simulink model "Capteur"  (R2019b)
settings: Solver=FixedStepAuto  StartTime=0.0  StopTime=1  FixedStep=0.0001  RelTol=1e-3
settings Model: Creator=Dell XPS  LastModifiedBy=jeanz
settings SolverCC: InitialStep=0.0001

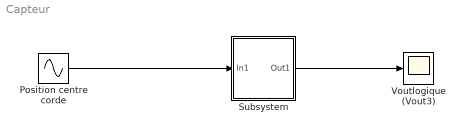
== system Capteur ==
  Position centre corde : Sin  Amplitude=0.1  Bias=2.415  Frequency=1256  SampleTime=0
  Subsystem : Subsystem
  Voutlogique (Vout3) : Scope
  wires:
  Position centre corde/1 -> Subsystem/1(In1)
  Subsystem/1(Out1) -> Voutlogique (Vout3)/1

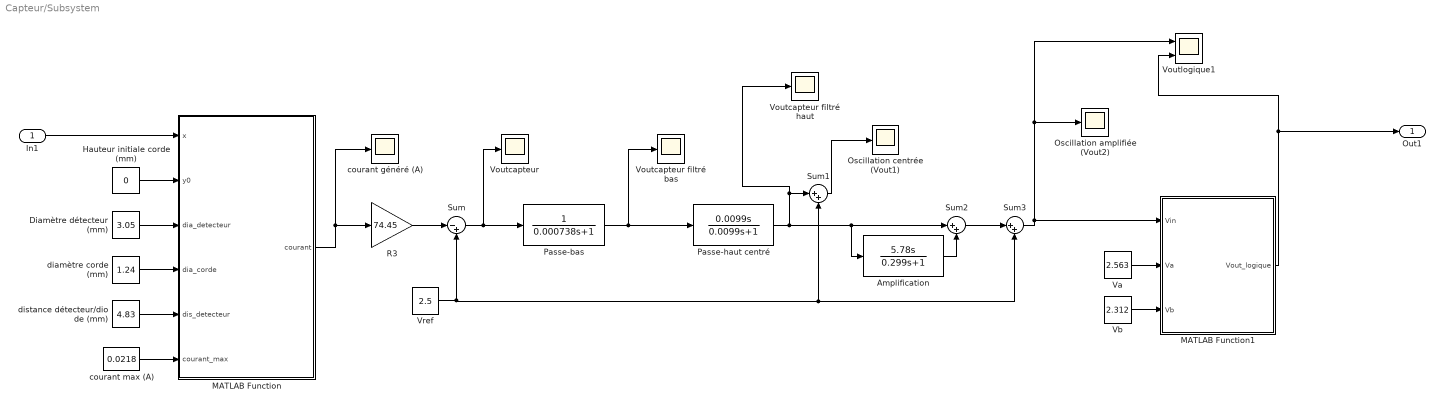
== system Capteur/Subsystem ==
  In1 : Inport
  "Amplification " : TransferFcn  Numerator=[5.78 0]  Denominator=[0.299 1]
  "Diamètre détecteur (mm) " : Constant  Value=3.05
  Hauteur initiale corde (mm) : Constant  Value=0
  MATLAB Function : MATLAB Function  TreatAsAtomicUnit=on
  MATLAB Function1 : MATLAB Function  TreatAsAtomicUnit=on
  "Oscillation amplifiée (Vout2) " : Scope
  Oscillation centrée (Vout1) : Scope
  Passe-bas : TransferFcn  Denominator=[0.000738 1]
  "Passe-haut centré " : TransferFcn  Numerator=[0.0099 0]  Denominator=[0.0099 1]
  R3 : Gain  Gain=74.45
  Sum : Sum  Inputs=|-+
  Sum1 : Sum  Inputs=|++
  Sum2 : Sum  Inputs=|++
  Sum3 : Sum  Inputs=|++
  "Va " : Constant  Value=2.563
  Vb : Constant  Value=2.312
  "Voutcapteur " : Scope
  Voutcapteur filtré bas : Scope
  Voutcapteur filtré haut : Scope
  Voutlogique1 : Scope  NumInputPorts=2
  "Vref " : Constant  Value=2.5
  "courant généré (A) " : Scope
  courant max (A) : Constant  Value=0.0218
  "diamètre corde (mm) " : Constant  Value=1.24
  "distance détecteur/diode (mm) " : Constant  Value=4.83
  Out1 : Outport
  wires:
  "Amplification "/1 -> Sum2/2
  "distance détecteur/diode (mm) "/1 -> MATLAB Function/5(dis_detecteur)
  Sum3/1 -> Voutlogique1/1, "Oscillation amplifiée (Vout2) "/1, MATLAB Function1/1(Vin)
  MATLAB Function/1(courant) -> R3/1, "courant généré (A) "/1
  "Vref "/1 -> Sum/2, Sum3/2, Sum1/2
  Sum/1 -> "Voutcapteur "/1, Passe-bas/1
  "Diamètre détecteur (mm) "/1 -> MATLAB Function/3(dia_detecteur)
  R3/1 -> Sum/1
  "Passe-haut centré "/1 -> Sum2/1, "Amplification "/1, Voutcapteur filtré haut/1, Sum1/1
  Vb/1 -> MATLAB Function1/3(Vb)
  Hauteur initiale corde (mm)/1 -> MATLAB Function/2(y0)
  Passe-bas/1 -> Voutcapteur filtré bas/1, "Passe-haut centré "/1
  Sum2/1 -> Sum3/1
  Sum1/1 -> Oscillation centrée (Vout1)/1
  MATLAB Function1/1(Vout_logique) -> Out1/1, Voutlogique1/2
  "Va "/1 -> MATLAB Function1/2(Va)
  "diamètre corde (mm) "/1 -> MATLAB Function/4(dia_corde)
  courant max (A)/1 -> MATLAB Function/6(courant_max)
  In1/1 -> MATLAB Function/1(x)

== matlab function Capteur/Subsystem/MATLAB Function1 ==
  data: Vin input; Vout_logique output; Va input; Vb input
function Vout_logique = fcn(Vin, Va, Vb)

Vout_logique = 0;
if Vin > Va && Vout_logique == 5
    Vout_logique = 0;
end
if Vin < Vb && Vout_logique == 0
    Vout_logique = 5;
end
end

== matlab function Capteur/Subsystem/MATLAB Function ==
  data: x input; y0 input; courant output; dia_detecteur input; dia_corde input; dis_detecteur input; courant_max input
function courant = fcn(x, y0, dia_detecteur, dia_corde, dis_detecteur, courant_max)

r = dia_detecteur/2;
angle_detection = atan((dia_detecteur/2)/dis_detecteur);
aire_detecteur = pi * (dia_detecteur/2)^2;


%distance centre corde
dis_centre_corde = sqrt(x^2 + y0^2);

%angle taille angulaire
delta = 2*asin(dia_corde/(2*dis_centre_corde));

%angle milieu corde
theta = atan(y0/x);

%angles par rapport au point d'observation de la corde (haut et bas)
delta_haut = theta + delta/2;
delta_bas = theta - delta/2;

%angles d'intérêts
if delta_haut >= angle_detection
    delta_haut = angle_detection;
end

if delta_bas <= -angle_detection
    delta_bas = -angle_detection;
end

%hauteur en y  sur le détecteur obstruée par corde
ydetecteur_haut = tan(delta_haut) *dis_detecteur;
ydetecteur_bas = tan(delta_bas) * dis_detecteur;
ydetecteur_haut = abs(ydetecteur_haut);
ydetecteur_bas = abs(ydetecteur_bas);



%aire sur détecteur obstruée par corde
aire_haut = r^2 * (asin(ydetecteur_haut/r) + (ydetecteur_haut/r) * sqrt(1- (ydetecteur_haut/r)^2));
aire_bas = r^2 * (asin(ydetecteur_bas/r) + (ydetecteur_bas/r) * sqrt(1- (ydetecteur_bas/r)^2));
aire_obstruee = aire_haut + aire_bas;

%courant
courant = ((aire_detecteur-aire_obstruee)/aire_detecteur) * courant_max;
return 
end
